simulink model "sgMdl_IO512_Loopback"  (R2024b)
settings: Solver=FixedStepAuto  StartTime=0.0  StopTime=inf  RelTol=1e-3  EnableMultiTasking=on
undefined symbols (not defined in the file): Abort, Biphase, FM1, Mark, NRZI, RS
libraries: speedgoatlib_IO512 x5, slrealtimeutilitieslib x4, simulink x1
Description:
  | IO512 - Loopback
settings Model: sg_rtwmakecfg_data=_sglibc_  ModifiedByFormat=Speedgoat  Creator=Speedgoat  LastModifiedBy=Speedgoat
settings SolverCC: ConcurrentTasks=on  AlgebraicLoopSolver=TrustRegion  PositivePriorityOrder=on
settings DataIOCC: LimitDataPoints=on  SaveFormat=Array  SignalLoggingSaveFormat=ModelDataLogs  ReturnWorkspaceOutputs=off
settings OptimizationCC: BlockReduction=off  OptimizeBlockIOStorage=off  BufferReuse=off  ReuseModelBlockBuffer=off  GlobalBufferReuse=off  ExpressionFolding=off  ExpressionDepthLimit=2147483647  LocalBlockOutputs=off  OptimizeDataStoreBuffers=off  BusAssignmentInplaceUpdate=off
settings DebuggingCC: UnderspecifiedInitializationDetection=Classic  MergeDetectMultiDrivingBlocksExec=none  SolverPrmCheckMsg=warning  TasksWithSamePriorityMsg=none  FcnCallInpInsideContextMsg=warning  UnconnectedInputMsg=warning  UnconnectedOutputMsg=warning  UnconnectedLineMsg=warning  StateNameClashWarn=warning  SFUnexpectedBacktrackingDiag=warning  SFNoUnconditionalDefaultTransitionDiag=warning  ArithmeticOperatorsInVariantConditions=warning
settings HardwareCC: ProdBitPerLong=64  ProdLongLongMode=on  ProdHWDeviceType=Intel->x86-64 (Linux 64)
settings ModelReferenceCC: EnableRefExpFcnMdlSchedulingChecks=on  PropagateSignalLabelsOutOfModel=off
settings SFSimCC: SimUseLocalCustomCode=off  CustomCodeUndefinedFunction=UseInterfaceOnly
settings RTWCC: Description=Speedgoat Real-Time Target Machine  SystemTargetFile=speedgoat.tlc  TemplateMakefile=slrealtime_default_tmf  RTWUseLocalCustomCode=off  Toolchain=Simulink Real-Time Toolchain  BuildConfiguration=Faster Runs  TargetLang=C++  GPUComputeCapability=3.5  DLArmComputeVersion=19.05
settings CodeAppCC: StateflowObjectComments=on
settings SimulinkRealTimeTargetCC: SubcomponentCodeInterfacePackaging=Reusable function  InstructionSetFMA=off  LogToMDFFile=off  SLRTFileLogMaxRuns=10  UseGCCFastMath=on
settings ConfigComp: CovMetricSettings=dw  CovSaveCumulativeToWorkspaceVar=on  CovSaveSingleToWorkspaceVar=on  CovExternalEMLEnable=off  CovSFcnEnable=off  CovBoundaryAbsTol=1.0e-5

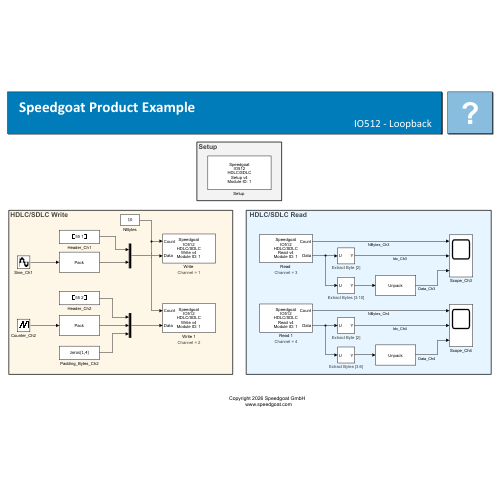
[thumbnail: Simulink's stored preview of the top-level diagram]
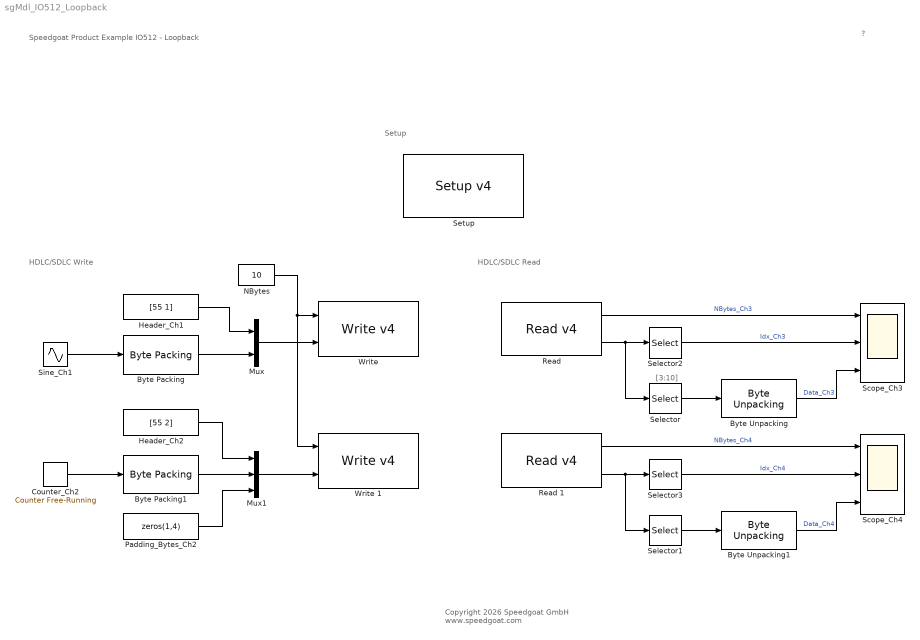
== system sgMdl_IO512_Loopback ==
  note: [3:10]
  note: Setup
  note: HDLC/SDLC Write
  note: HDLC/SDLC Read
  note: Speedgoat Product Example
      | IO512 - Loopback
  note: ?
  note: Copyright 2026 Speedgoat GmbH
      |  www.speedgoat.com
  Byte Packing : slrealtimeutilitieslib/Byte Packing  MaskPackedDataType=uint8  MaskUnpackedDataTypes={'double'}  MaskAlignment=1
  Byte Packing1 : slrealtimeutilitieslib/Byte Packing  MaskPackedDataType=uint8  MaskUnpackedDataTypes={'uint32'}  MaskAlignment=1
  Byte Unpacking : slrealtimeutilitieslib/Byte Unpacking  MaskUnpackedDataTypes={'double'}  MaskUnpackedDataSizes={[1]}  MaskAlignment=1
  Byte Unpacking1 : slrealtimeutilitieslib/Byte Unpacking  MaskUnpackedDataTypes={'uint32'}  MaskUnpackedDataSizes={[1]}  MaskAlignment=1
  Counter_Ch2 : simulink/Sources/Counter Free-Running  NumBits=32  tsamp=0.01
  Header_Ch1 : Constant  Value=[55 1]  OutDataTypeStr=Inherit: Inherit via back propagation  SampleTime=0.01
  Header_Ch2 : Constant  Value=[55 2]  OutDataTypeStr=Inherit: Inherit via back propagation  SampleTime=0.01
  Mux : Mux  Inputs=2
  Mux1 : Mux  Inputs=3
  NBytes : Constant  Value=10  OutDataTypeStr=Inherit: Inherit via back propagation  SampleTime=0.01
  Padding_Bytes_Ch2 : Constant  Value=zeros(1,4)  OutDataTypeStr=Inherit: Inherit via back propagation  SampleTime=0.01
  "Read " : speedgoatlib_IO512/Read v4   parModuleId=1  parCh=3  parTs=0.01  parFifoSize=20  parPciSlot=-1
      settings: AttributesFormatString=Channel = %<parCh>  SourceProductName=Simulink Real-Time: Speedgoat I/O Blockset
  Read 1 : speedgoatlib_IO512/Read v4   parModuleId=1  parCh=4  parTs=0.01  parFifoSize=20  parPciSlot=-1
      settings: AttributesFormatString=Channel = %<parCh>  SourceProductName=Simulink Real-Time: Speedgoat I/O Blockset
  Scope_Ch3 : Scope  NumInputPorts=3
  Scope_Ch4 : Scope  NumInputPorts=3
  Selector : Selector  InputPortWidth=20  IndexOptions=Index vector (dialog)  Indices=[3:10]  OutputSizes=1
      settings: AttributesFormatString=Extract Bytes %<Indices>
  Selector1 : Selector  InputPortWidth=20  IndexOptions=Index vector (dialog)  Indices=[3:6]  OutputSizes=1
      settings: AttributesFormatString=Extract Bytes %<Indices>
  Selector2 : Selector  InputPortWidth=20  IndexOptions=Index vector (dialog)  Indices=[2]  OutputSizes=1
      settings: AttributesFormatString=Extract Byte %<Indices>
  Selector3 : Selector  InputPortWidth=20  IndexOptions=Index vector (dialog)  Indices=[2]  OutputSizes=1
      settings: AttributesFormatString=Extract Byte %<Indices>
  "Setup " : speedgoatlib_IO512/Setup v4   parModuleId=1  parPciSlot=-1  parTransceiver1=RS-422 / RS-485  parTransceiver2=RS-422 / RS-485  parTransceiver3=RS-422 / RS-485  parTransceiver4=RS-422 / RS-485  parMode1=DTE  parChFreq1=5e6  parEncoding1=Biphase-Mark (FM1)  parDataSize1=10  parUnderrunResp1=Abort (01111111)  parTxIdle1=Flags  parTxParity1=No parity  parFlagShareZero1=off  parTxPreamble1=None  parTxPreambleLen1=8 Bits  parTxCharLen1=8  parTxCrc1=No CRC  parTxClkSrc1=Internal Clock  parRxFifoThresh1=15  parRxSwFifoSize1=20  parRxParity1=No Parity  parRxCharLen1=8  parRxAddrCtl1=No Address or Control field handling  parRxSync1=0  parRxCrc1=No CRC  parRxClkSrc1=Internal Clock  parTermResist1=off  parMode2=DTE  parChFreq2=115200  parEncoding2=NRZI-Mark  parDataSize2=10  parUnderrunResp2=Abort (01111111)  parTxIdle2=Flags  parTxParity2=No parity  parFlagShareZero2=off  parTxPreamble2=None  parTxPreambleLen2=8 Bits  parTxCharLen2=8  parTxCrc2=No CRC  parTxClkSrc2=RxC Input Pin  parRxFifoThresh2=15  parRxSwFifoSize2=20  parRxParity2=No Parity  parRxCharLen2=8  parRxAddrCtl2=No Address or Control field handling  parRxSync2=0  parRxCrc2=No CRC  parRxClkSrc2=RxC Input Pin  parTermResist2=off  parMode3=DCE  parChFreq3=5e6  parEncoding3=Biphase-Mark (FM1)  parDataSize3=10  parUnderrunResp3=Abort (01111111)  parTxIdle3=Flags  parTxParity3=No parity  parFlagShareZero3=off  parTxPreamble3=None  parTxPreambleLen3=8 Bits  parTxCharLen3=8  parTxCrc3=No CRC  parTxClkSrc3=Internal Clock  parRxFifoThresh3=15  parRxSwFifoSize3=20  parRxParity3=No Parity  parRxCharLen3=8  parRxAddrCtl3=No Address or Control field handling  parRxSync3=0  parRxCrc3=No CRC  parRxClkSrc3=Internal Clock  parTermResist3=off  parMode4=DCE  parChFreq4=115200  parEncoding4=NRZI-Mark  parDataSize4=10  parUnderrunResp4=Abort (01111111)  parTxIdle4=Flags  parTxParity4=No parity  parFlagShareZero4=off  parTxPreamble4=None  parTxPreambleLen4=8 Bits  parTxCharLen4=8  parTxCrc4=No CRC  parTxClkSrc4=Internal Clock  parRxFifoThresh4=15  parRxSwFifoSize4=20  parRxParity4=No Parity  parRxCharLen4=8  parRxAddrCtl4=No Address or Control field handling  parRxSync4=0  parRxCrc4=No CRC  parRxClkSrc4=RxC Input Pin  parTermResist4=off
      settings: SourceProductName=Simulink Real-Time: Speedgoat I/O Blockset
  Sine_Ch1 : Sin  Amplitude=10  Frequency=2*pi  SampleTime=0.01
  "Write " : speedgoatlib_IO512/Write v4   parModuleId=1  parCh=1  parTs=-1  parMaxCnt=10  parPciSlot=-1
      settings: AttributesFormatString=Channel = %<parCh>  SourceProductName=Simulink Real-Time: Speedgoat I/O Blockset
  Write 1 : speedgoatlib_IO512/Write v4   parModuleId=1  parCh=2  parTs=-1  parMaxCnt=10  parPciSlot=-1
      settings: AttributesFormatString=Channel = %<parCh>  SourceProductName=Simulink Real-Time: Speedgoat I/O Blockset
  wires:
  Byte Packing/1 -> Mux/2
  Header_Ch1/1 -> Mux/1
  Mux/1 -> "Write "/2
  NBytes/1 -> Write 1/1, "Write "/1
  "Read "/1 -> Scope_Ch3/1  "NBytes_Ch3"
  Sine_Ch1/1 -> Byte Packing/1
  Mux1/1 -> Write 1/2
  Header_Ch2/1 -> Mux1/1
  Byte Packing1/1 -> Mux1/2
  Counter_Ch2/1 -> Byte Packing1/1
  Padding_Bytes_Ch2/1 -> Mux1/3
  "Read "/2 -> Selector2/1, Selector/1
  Selector/1 -> Byte Unpacking/1
  Read 1/1 -> Scope_Ch4/1  "NBytes_Ch4"
  Selector1/1 -> Byte Unpacking1/1
  Read 1/2 -> Selector3/1, Selector1/1
  Byte Unpacking/1 -> Scope_Ch3/3  "Data_Ch3"
  Selector2/1 -> Scope_Ch3/2  "Idx_Ch3"
  Byte Unpacking1/1 -> Scope_Ch4/3  "Data_Ch4"
  Selector3/1 -> Scope_Ch4/2  "Idx_Ch4"
